simulink model "kinematicCar"  (R2025b)
settings: Solver=VariableStepAuto  StartTime=0.0  StopTime=10.0  RelTol=1e-3
settings Model: Creator=sprinkle  LastModifiedBy=sprinkle

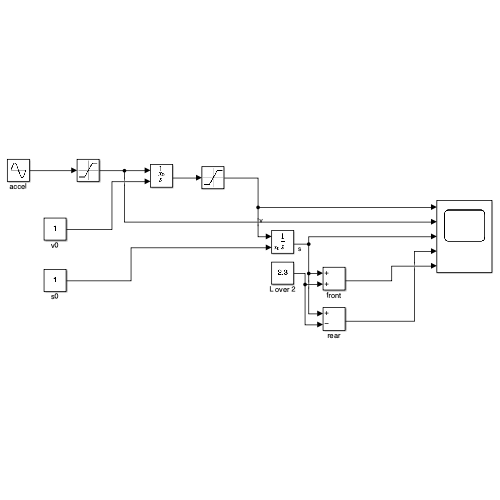
[thumbnail: Simulink's stored preview of the top-level diagram]
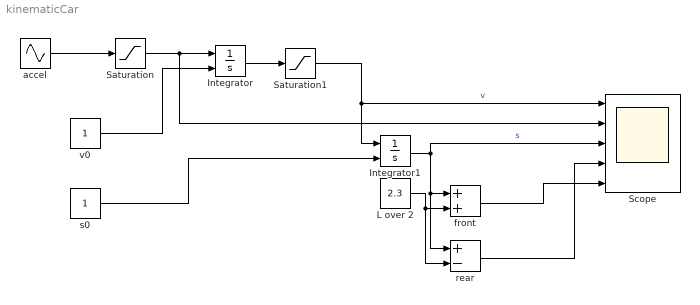
== system kinematicCar ==
  Integrator : Integrator  InitialConditionSource=external
  Integrator1 : Integrator  InitialConditionSource=external
  L over 2 : Constant  Value=2.3
  Saturation : Saturate  UpperLimit=1.5  LowerLimit=-3.5
  Saturation1 : Saturate  UpperLimit=30  LowerLimit=0
  Scope : Scope  NumInputPorts=5
      settings: ActiveDisplayYMinimum=-6.4319436824788268  ActiveDisplayYMaximum=22.887493142309445
  accel : Sin  Amplitude=5  SampleTime=0
  front : Sum
  rear : Sum  Inputs=+-
  s0 : Constant
  v0 : Constant
  wires:
  accel/1 -> Saturation/1
  Integrator/1 -> Saturation1/1
  v0/1 -> Integrator/2
  s0/1 -> Integrator1/2
  Integrator1/1 -> rear/1, front/1, Scope/3  "s"
  Saturation/1 -> Scope/2, Integrator/1
  Saturation1/1 -> Integrator1/1, Scope/1  "v"
  L over 2/1 -> rear/2, front/2
  front/1 -> Scope/5
  rear/1 -> Scope/4
